simulink model "gm_ldpc_dvbs2_model_v2_fil"  (R2020b)
settings: Solver=FixedStepDiscrete  StartTime=0.0  StopTime=360*135 + 16200  RelTol=1e-3
libraries: simulink x4, hdlsllib x4, fillib x1
settings Model: Creator=wardo  LastModifiedBy=wardo
settings DataIOCC: LimitDataPoints=on  SaveOutput=off  SaveTime=off
settings OptimizationCC: BlockReduction=off  ConditionallyExecuteInputs=off  DefaultParameterBehavior=Inlined  LifeSpan=inf
settings DebuggingCC: AlgebraicLoopMsg=error  InheritedTsInSrcMsg=none  SingleTaskRateTransMsg=error  AllowSymbolicDim=off  StrictBusMsg=ErrorOnBusTreatedAsVector  SFUnexpectedBacktrackingDiag=warning  SFNoUnconditionalDefaultTransitionDiag=warning  SFExecutionAtInitializationDiag=none  ArithmeticOperatorsInVariantConditions=warning
settings HardwareCC: ProdBitPerPointer=32  ProdBitPerSizeT=32  ProdBitPerPtrDiffT=32  ProdLargestAtomicFloat=None  ProdIntDivRoundTo=Undefined  ProdEndianess=Unspecified  ProdWordSize=32  ProdHWDeviceType=ASIC/FPGA->ASIC/FPGA  ProdEqTarget=off
settings SFSimCC: SimUseLocalCustomCode=off  CustomCodeUndefinedFunction=UseInterfaceOnly
settings RTWCC: RTWUseLocalCustomCode=off
settings CodeAppCC: StateflowObjectComments=on
settings GRTTargetCC: TargetLangStandard=C89/C90 (ANSI)
settings ConfigComp: CovScope=ReferencedModels  CovMetricSettings=dw  CovSaveCumulativeToWorkspaceVar=on  CovSaveSingleToWorkspaceVar=on  CovExternalEMLEnable=off  CovSFcnEnable=off

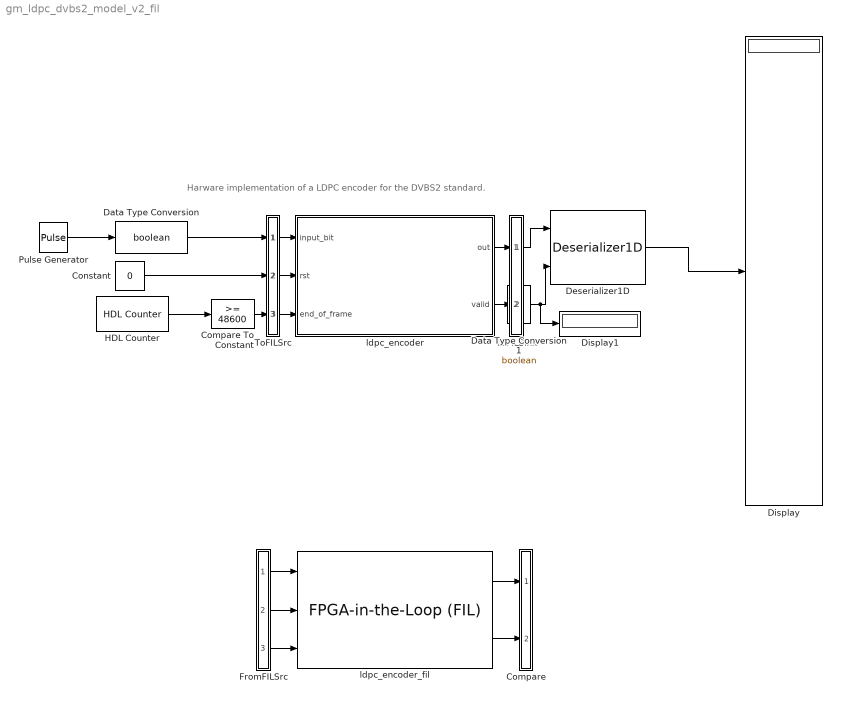
== system gm_ldpc_dvbs2_model_v2_fil ==
  note: Harware implementation of a LDPC encoder for the DVBS2 standard.
  Compare : Subsystem
      mask Display: disp('')
  Compare To Constant : simulink/Logic and Bit Operations/Compare To Constant  relop=>=  const=48600  OutDataTypeStr=boolean
  Constant : Constant  Value=0  OutDataTypeStr=boolean
  Data Type Conversion : DataTypeConversion  OutDataTypeStr=boolean
  Data Type Conversion1 : DataTypeConversion  OutDataTypeStr=boolean
  Deserializer1D : hdlsllib/HDL Operations/Deserializer1D  Ratio=16200  IdleCycles=0  InitialCondition=0  startIn=off  validIn=on  validOut=off  inputDataDimensions=-1  inputSampleTime=-1  inputSignalType=auto
      settings: SourceProductBaseCode=SL
  Display : Display
  Display1 : Display
  FromFILSrc : Subsystem
      mask Display: disp('')
  HDL Counter : hdlsllib/Sources/HDL Counter  CountType=Count limited  CountInit=1  CountStep=1  CountMax=48600  CountFromType=Initial value  CountFrom=1  CountResetPort=off  CountLoadPort=off  CountEnbPort=off  CountDirPort=off  CountDataType=Unsigned  CountWordLen=16  CountFracLen=0  CountSampTime=1
  Pulse Generator : DiscretePulseGenerator  PulseType=Time based  PulseWidth=50
  ToFILSink : Subsystem
      mask Display: disp('')
  ToFILSrc : Subsystem
      mask Display: disp('')
  ldpc_encoder : Subsystem
  ldpc_encoder_fil : fillib/FPGA-in-the-Loop (FIL)  ForceInterfaceUpdate=0.90579
      settings: SourceProductBaseCode=ES,HD
  wires:
  Pulse Generator/1 -> Data Type Conversion/1
  HDL Counter/1 -> Compare To Constant/1
  Deserializer1D/1 -> Display/1
  Data Type Conversion1/1 -> Deserializer1D/2, Display1/1
  ToFILSrc/1(out1) -> ldpc_encoder/1(input_bit)
  ToFILSrc/2(out2) -> ldpc_encoder/2(rst)
  ToFILSrc/3(out3) -> ldpc_encoder/3(end_of_frame)
  ldpc_encoder/1(out) -> ToFILSink/1(in1)
  ldpc_encoder/2(valid) -> ToFILSink/2(in2)
  Data Type Conversion/1 -> ToFILSrc/1(in1)
  Constant/1 -> ToFILSrc/2(in2)
  Compare To Constant/1 -> ToFILSrc/3(in3)
  ToFILSink/1(out1) -> Deserializer1D/1
  ToFILSink/2(out2) -> Data Type Conversion1/1
  FromFILSrc/1(out1) -> ldpc_encoder_fil/1
  FromFILSrc/2(out2) -> ldpc_encoder_fil/2
  FromFILSrc/3(out3) -> ldpc_encoder_fil/3
  ldpc_encoder_fil/1 -> Compare/1(in1)
  ldpc_encoder_fil/2 -> Compare/2(in2)

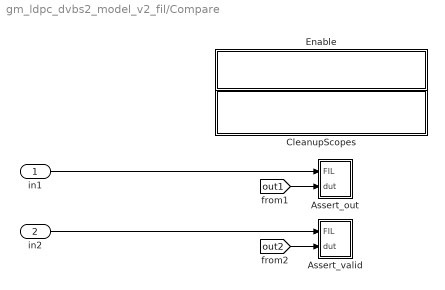
== system gm_ldpc_dvbs2_model_v2_fil/Compare ==
  in1 : Inport
  in2 : Inport  Port=2
  Assert_out : Subsystem
  Assert_valid : Subsystem
  CleanupScopes : Subsystem
      settings: OpenFcn=|
      | blkName = gcb; %self block
      | idx = regexp(blkName, '/CleanupScopes$', 'once');
      | blkParent = blkName(1:idx-1);
      | blks=find_system(blkParent, 'LookUnderMasks', 'all','blocktype', 'Scope');
      | for itr = 1:length(blks)
      | 	 hScopeCfg = get_param(blks{itr},'ScopeConfiguration');
      | 	 hScopeCfg.Visible = ~ hScopeCfg.Visible;
      | end
      | drawnow;
      mask Display: fprintf(message('hdlcoder:cosim:vnl_dblclick').getString());
  Enable : Subsystem
      settings: OpenFcn=|
      | blkName = gcb;
      | idx = regexp(blkName, '/Enable$', 'once');
      | blkParent = blkName(1:idx-1);
      | blks=find_system(blkParent, 'LookUnderMasks', 'all','blocktype', 'Assertion');
      | e = get_param(blks{1}, 'Enabled');
      | if strcmp(e, 'on'), f= 'off';, else, f = 'on';, end
      | for ii=1:length(blks), set_param(blks{ii}, 'Enabled', f);, end
      | set_param(gcb, 'MaskDisplay',['fprintf(message(''hdlcoder:cosim:vnl_dblclick_assertions'',','''',upper(e),'''',').getString())']);
      mask Display: fprintf(message('hdlcoder:cosim:vnl_dblclick_assertions','OFF').getString());
  wires:
  in1/1 -> Assert_out/1(FIL)
  [out1] -> Assert_out/2(dut)
  in2/1 -> Assert_valid/1(FIL)
  [out2] -> Assert_valid/2(dut)

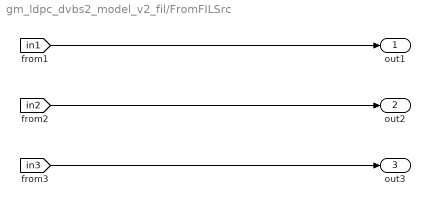
== system gm_ldpc_dvbs2_model_v2_fil/FromFILSrc ==
  out1 : Outport
  out2 : Outport  Port=2
  out3 : Outport  Port=3
  wires:
  [in1] -> out1/1
  [in2] -> out2/1
  [in3] -> out3/1

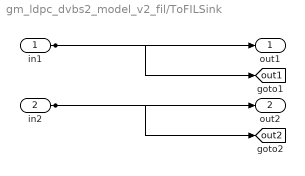
== system gm_ldpc_dvbs2_model_v2_fil/ToFILSink ==
  in1 : Inport
  in2 : Inport  Port=2
  out1 : Outport
  out2 : Outport  Port=2
  tag scope: out1=global, out2=global
  wires:
  in1/1 -> out1/1, [out1]
  in2/1 -> out2/1, [out2]

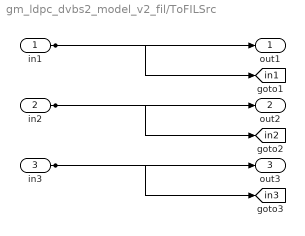
== system gm_ldpc_dvbs2_model_v2_fil/ToFILSrc ==
  in1 : Inport
  in2 : Inport  Port=2
  in3 : Inport  Port=3
  out1 : Outport
  out2 : Outport  Port=2
  out3 : Outport  Port=3
  tag scope: in1=global, in2=global, in3=global
  wires:
  in1/1 -> out1/1, [in1]
  in2/1 -> out2/1, [in2]
  in3/1 -> out3/1, [in3]

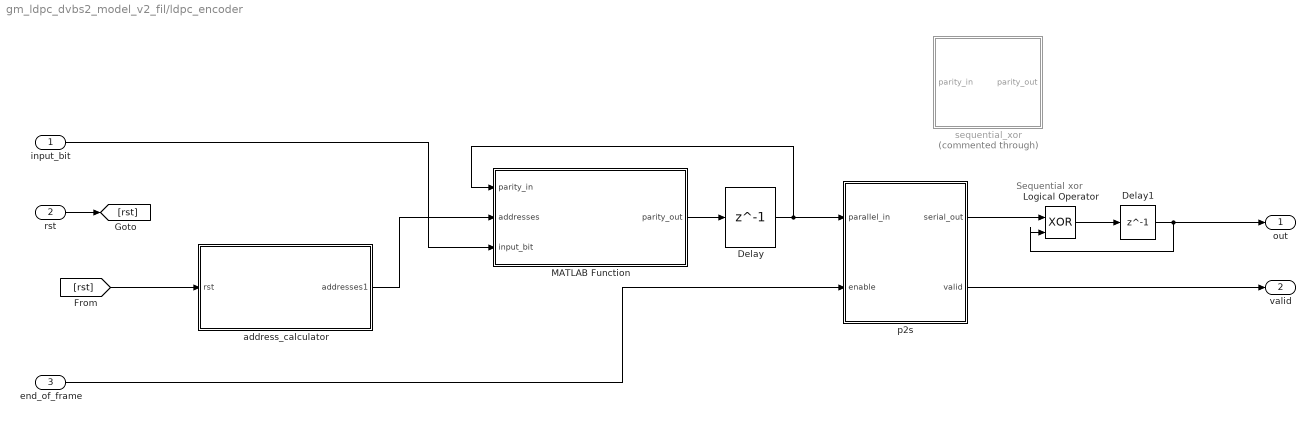
== system gm_ldpc_dvbs2_model_v2_fil/ldpc_encoder ==
  note: Sequential xor
  input_bit : Inport
  rst : Inport  Port=2
  end_of_frame : Inport  Port=3
  Delay : Delay  DelayLength=1  InitialCondition=[zeros(16200, 1); 1]
  Delay1 : Delay  DelayLength=1
  Logical Operator : Logic  Operator=XOR  IconShape=distinctive  AllPortsSameDT=off  OutDataTypeStr=fixdt(0,1, 0)
  MATLAB Function : MATLAB Function  TreatAsAtomicUnit=on
  address_calculator : Subsystem
  p2s : MATLAB Function  TreatAsAtomicUnit=on  mask{input_length=16200}
  sequential_xor : MATLAB Function  Commented=through  TreatAsAtomicUnit=on  mask{num_parity_bits=16200}
  out : Outport  VectorParamsAs1DForOutWhenUnconnected=off
  valid : Outport  Port=2  VectorParamsAs1DForOutWhenUnconnected=off
  wires:
  input_bit/1 -> MATLAB Function/3(input_bit)
  rst/1 -> [rst]
  MATLAB Function/1(parity_out) -> Delay/1
  Delay/1 -> MATLAB Function/1(parity_in), p2s/1(parallel_in)
  address_calculator/1(addresses1) -> MATLAB Function/2(addresses)
  [rst] -> address_calculator/1(rst)
  end_of_frame/1 -> p2s/2(enable)
  p2s/2(valid) -> valid/1
  p2s/1(serial_out) -> Logical Operator/1
  Logical Operator/1 -> Delay1/1
  Delay1/1 -> Logical Operator/2, out/1

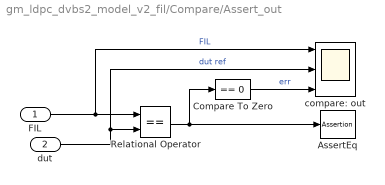
== system gm_ldpc_dvbs2_model_v2_fil/Compare/Assert_out ==
  FIL : Inport
  dut : Inport  Port=2
  AssertEq : Assertion  StopWhenAssertionFail=off
  Compare To Zero : simulink/Logic and Bit Operations/Compare To Zero  relop===  OutDataTypeStr=boolean
  Relational Operator : RelationalOperator  Operator===  OutDataTypeStr=boolean  RndMeth=Nearest
  compare: out : Scope  NumInputPorts=3
  wires:
  Compare To Zero/1 -> compare: out/3  "err"
  Relational Operator/1 -> Compare To Zero/1, AssertEq/1
  FIL/1 -> compare: out/1, Relational Operator/1  "FIL"
  dut/1 -> compare: out/2, Relational Operator/2  "dut ref"

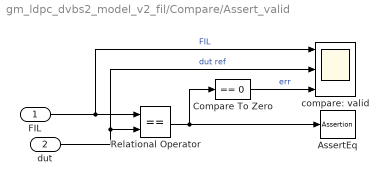
== system gm_ldpc_dvbs2_model_v2_fil/Compare/Assert_valid ==
  FIL : Inport
  dut : Inport  Port=2
  AssertEq : Assertion  StopWhenAssertionFail=off
  Compare To Zero : simulink/Logic and Bit Operations/Compare To Zero  relop===  OutDataTypeStr=boolean
  Relational Operator : RelationalOperator  Operator===  OutDataTypeStr=boolean  RndMeth=Nearest
  compare: valid : Scope  NumInputPorts=3
  wires:
  Compare To Zero/1 -> compare: valid/3  "err"
  Relational Operator/1 -> Compare To Zero/1, AssertEq/1
  FIL/1 -> compare: valid/1, Relational Operator/1  "FIL"
  dut/1 -> compare: valid/2, Relational Operator/2  "dut ref"

== system gm_ldpc_dvbs2_model_v2_fil/Compare/CleanupScopes ==

== system gm_ldpc_dvbs2_model_v2_fil/Compare/Enable ==

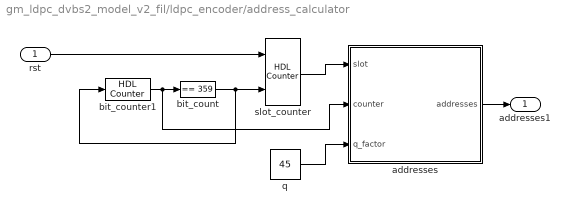
== system gm_ldpc_dvbs2_model_v2_fil/ldpc_encoder/address_calculator ==
  rst : Inport
  addresses : MATLAB Function  TreatAsAtomicUnit=on  mask{bit_addresses=uint16([[0 6385 7901 14611 13389 11200 3252 5243 2504 2722 821 7374]; [1 11359 2698 357 13824 12772 7244 6752 15310 852 2001 11417]; [2 7862 7977 6321 13612 12197 14449 15137 13860 1708 6399 13444]; [3 1560 11804 6975 13292 3646 3812 8772 7306 5795 14327 7866]; [4 7626 11407 14599 9689 1628 2113 10809 9283 1230 15241 4870]; [5 1610 5699 15876 9446 12515 1400 6303 5411 14181 13925 7358]; [6 4059 8836 3405 7853 7992 15336 5970 10368 10278 9675 4651]; [7 4441 3963 9153 2109 12683 7459 12030 12221 629 15212 406]; [8 6007 8411 5771 3497 543 14202 875 9186 6235 13908 3563]; [9 3232 6625 4795 546 9781 2071 7312 3399 7250 4932 12652]; [10 8820 10088 11090 7069 6585 13134 10158 7183 488 7455 9238]; [11 1903 10818 119 215 7558 11046 10615 11545 14784 7961 15619]; [12 3655 8736 4917 15874 5129 2134 15944 14768 7150 2692 1469]; [13 8316 3820 505 8923 6757 806 7957 4216 15589 13244 2622]; [14 14463 4852 15733 3041 11193 12860 13673 8152 6551 15108 8758]; [15 3149 11981 16200 16200 16200 16200 16200 16200 16200 16200 16200]; [16 13416 6906 16200 16200 16200 16200 16200 16200 16200 16200 16200]; [17 13098 13352 16200 16200 16200 16200 16200 16200 16200 16200 16200]; [18 2009 14460 16200 16200 16200 16200 16200 16200 16200 16200 16200]; [19 7207 4314 16200 16200 16200 16200 16200 16200 16200 16200 16200]; [20 3312 3945 16200 16200 16200 16200 16200 16200 16200 16200 16200]; [21 4418 6248 16200 16200 16200 16200 16200 16200 16200 16200 16200]; [22 2669 13975 16200 16200 16200 16200 16200 16200 16200 16200 16200]; [23 7571 9023 16200 16200 16200 16200 16200 16200 16200 16200 16200]; [24 14172 2967 16200 16200 16200 16200 16200 16200 16200 16200 16200]; [25 7271 7138 16200 16200 16200 16200 16200 16200 16200 16200 16200]; [26 6135 13670 16200 16200 16200 16200 16200 16200 16200 16200 16200]; [27 7490 14559 16200 16200 16200 16200 16200 16200 16200 16200 16200]; [28 8657 2466 16200 16200 16200 16200 16200 16200 16200 16200 16200]; [29 8599 12834 16200 16200 16200 16200 16200 16200 16200 16200 16200]; [30 3470 3152 16200 16200 16200 16200 16200 16200 16200 16200 16200]; [31 13917 4365 16200 16200 16200 16200 16200 16200 16200 16200 16200]; [32 6024 13730 16200 16200 16200 16200 16200 16200 16200 16200 16200]; [33 10973 14182 16200 16200 16200 16200 16200 16200 16200 16200 16200]; [34 2464 13167 16200 16200 16200 16200 16200 16200 16200 16200 16200]; [35 5281 15049 16200 16200 16200 16200 16200 16200 16200 16200 16200]; [36 1103 1849 16200 16200 16200 16200 16200 16200 16200 16200 16200]; [37 2058 1069 16200 16200 16200 16200 16200 16200 16200 16200 16200]; [38 9654 6095 16200 16200 16200 16200 16200 16200 16200 16200 16200]; [39 14311 7667 16200 16200 16200 16200 16200 16200 16200 16200 16200]; [40 15617 8146 16200 16200 16200 16200 16200 16200 16200 16200 16200]; [41 4588 11218 16200 16200 16200 16200 16200 16200 16200 16200 16200]; [42 13660 6243 16200 16200 16200 16200 16200 16200 16200 16200 16200]; [43 8578 7874 16200 16200 16200 16200 16200 16200 16200 16200 16200]; [44 11741 2686 16200 16200 16200 16200 16200 16200 16200 16200 16200]; [0 1022 1264 16200 16200 16200 16200 16200 16200 16200 16200 16200]; [1 12604 9965 16200 16200 16200 16200 16200 16200 16200 16200 16200]; [2 8217 2707 16200 16200 16200 16200 16200 16200 16200 16200 16200]; [3 3156 11793 16200 16200 16200 16200 16200 16200 16200 16200 16200]; [4 354 1514 16200 16200 16200 16200 16200 16200 16200 16200 16200]; [5 6978 14058 16200 16200 16200 16200 16200 16200 16200 16200 16200]; [6 7922 16079 16200 16200 16200 16200 16200 16200 16200 16200 16200]; [7 15087 12138 16200 16200 16200 16200 16200 16200 16200 16200 16200]; [8 5053 6470 16200 16200 16200 16200 16200 16200 16200 16200 16200]; [9 12687 14932 16200 16200 16200 16200 16200 16200 16200 16200 16200]; [10 15458 1763 16200 16200 16200 16200 16200 16200 16200 16200 16200]; [11 8121 1721 16200 16200 16200 16200 16200 16200 16200 16200 16200]; [12 12431 549 16200 16200 16200 16200 16200 16200 16200 16200 16200]; [13 4129 7091 16200 ...(+5412 chars)]]);, num_parity_bits=16200}
  bit_count : simulink/Logic and Bit Operations/Compare To Constant  relop===  const=359  OutDataTypeStr=boolean
  bit_counter1 : hdlsllib/Sources/HDL Counter  CountType=Count limited  CountInit=0  CountStep=1  CountMax=359  CountFromType=Initial value  CountFrom=0  CountResetPort=on  CountLoadPort=off  CountEnbPort=off  CountDirPort=off  CountDataType=Unsigned  CountWordLen=9  CountFracLen=0  CountSampTime=1
  q : Constant  Value=45  OutDataTypeStr=uint8  SampleTime=-1
  slot_counter : hdlsllib/Sources/HDL Counter  CountType=Count limited  CountInit=1  CountStep=1  CountMax=135  CountFromType=Initial value  CountFrom=1  CountResetPort=on  CountLoadPort=off  CountEnbPort=on  CountDirPort=off  CountDataType=Unsigned  CountWordLen=8  CountFracLen=0  CountSampTime=1
  addresses1 : Outport
  wires:
  addresses/1(addresses) -> addresses1/1
  bit_counter1/1 -> addresses/2(counter), bit_count/1
  bit_count/1 -> bit_counter1/1, slot_counter/2
  q/1 -> addresses/3(q_factor)
  rst/1 -> slot_counter/1
  slot_counter/1 -> addresses/1(slot)

== matlab function gm_ldpc_dvbs2_model_v2_fil/ldpc_encoder/sequential_xor ==
  settings: fimath=fimath('RoundingMethod', 'Floor','OverflowAction', 'Wrap','ProductMode', 'FullPrecision', 'SumMode', 'FullPrecision')
  data: parity_in input; parity_out output; num_parity_bits parameter uint16
function parity_out = sequential_xor(parity_in, num_parity_bits)
%#codegen

parity_out = fi(zeros(num_parity_bits, 1), 0, 1, 0);
parity_out(1) = parity_in(1);
for i = 2:num_parity_bits
    parity_out(i) = xor(parity_in(i), parity_out(i-1));
end

== matlab function gm_ldpc_dvbs2_model_v2_fil/ldpc_encoder/address_calculator/addresses ==
  settings: fimath=fimath('RoundingMethod', 'Floor','OverflowAction', 'Wrap','ProductMode', 'FullPrecision', 'SumMode', 'FullPrecision')
  data: slot input; counter input; q_factor input; addresses output uint16; bit_addresses parameter uint16; num_parity_bits parameter uint16
function addresses = address_generator(slot, counter, q_factor, bit_addresses, num_parity_bits)
%#codegen
buffer = uint16(bit_addresses(slot, :) + counter*q_factor);
addresses = buffer - uint16(num_parity_bits) .* uint16(buffer >= num_parity_bits);

== matlab function gm_ldpc_dvbs2_model_v2_fil/ldpc_encoder/p2s ==
  settings: fimath=fimath('RoundingMethod', 'Floor','OverflowAction', 'Wrap','ProductMode', 'FullPrecision', 'SumMode', 'FullPrecision')
  data: parallel_in input; serial_out output fixdt(0,1,0); enable input; input_length parameter uint16; valid output
function [serial_out, valid] = p2s_buffer(parallel_in, enable, input_length)
%#codegen

state_iddle   = 0;
state_reading = 1;

persistent moore_state_machine;
if isempty(moore_state_machine)
    moore_state_machine = fi(0, 0, 1, 0);
end

persistent counter;
if isempty(counter)
    counter = fi(1, 0, 16, 0);
end

persistent buffer;
if isempty(buffer)
    buffer = parallel_in;
end

switch moore_state_machine
    case state_iddle
        serial_out = fi(0, 0, 1, 0);
        valid      = fi(0, 0, 1, 0);
        if enable
            moore_state_machine(1) = state_reading;
            buffer = parallel_in;
            serial_out          = buffer(counter);
            counter             = fi(counter + 1, 0, 16, 0);
            valid               = fi(1, 0, 1, 0);
        end
    case state_reading
        serial_out = buffer(counter);
        counter    = fi(counter + 1, 0, 16, 0);
        valid      = fi(1, 0, 1, 0);
        if(counter > input_length)
            moore_state_machine(1) = state_iddle;
        end
    otherwise
        serial_out = fi(0, 0, 1, 0);
        valid      = fi(0, 0, 1, 0);
end

== matlab function gm_ldpc_dvbs2_model_v2_fil/ldpc_encoder/MATLAB Function ==
  settings: fimath=fimath('RoundingMethod', 'Floor','OverflowAction', 'Wrap','ProductMode', 'FullPrecision', 'SumMode', 'FullPrecision')
  data: parity_in input fixdt(0,1,0); parity_out output fixdt(0,1,0); addresses input; input_bit input
function parity_out = select_and_xor(parity_in, addresses, input_bit)
%#codegen

parity_out = parity_in;
parity_out(addresses+1) = xor(parity_in(addresses+1), input_bit);
